simulink model "Key_signal_process"  (R2021a)
settings: configuration reference "AION_IDS_Speedgoat" (kept outside this file)
undefined symbols (not defined in the file): original_value_current, original_value_previous, original_value_queue, processed_value_current, processed_value_previous, processed_value_queue, refitted_value_current, refitted_value_previous, refitted_value_queue, Validation
libraries: simulink x5
settings Model: DataDictionary=Key_Signal_Process.sldd  Creator=xinrui  LastModifiedBy=Administrator
settings ConfigSetRef: SourceName=AION_IDS_Speedgoat

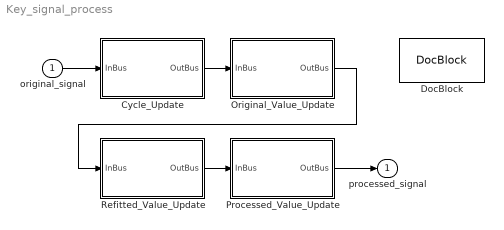
== system Key_signal_process ==
  original_signal : Inport  OutDataTypeStr=Bus: Key_Signal_Info  PortDimensions=1
  Cycle_Update : Subsystem
  DocBlock : simulink/Model-Wide Utilities/DocBlock  DocumentType=HTML  mask(DocBlock){}
      mask Display:
      | plot([.8 0 0 1 1 .8 .8 1],[1 1 0 0 .8 1 .8 .8]);
      | text(.5,.6,'CHANGELOG','horizontalalignment','center');
      | text(.95,.05,get_param(gcb,'DocumentType'),'verticalalignment','bottom','horizontalalignment','right');
  Original_Value_Update : Subsystem
  Processed_Value_Update : Subsystem
  Refitted_Value_Update : Subsystem
  processed_signal : Outport  OutDataTypeStr=Bus: Key_Signal_Info  PortDimensions=1
  wires:
  Refitted_Value_Update/1(OutBus) -> Processed_Value_Update/1(InBus)
  Original_Value_Update/1(OutBus) -> Refitted_Value_Update/1(InBus)
  original_signal/1 -> Cycle_Update/1(InBus)
  Processed_Value_Update/1(OutBus) -> processed_signal/1
  Cycle_Update/1(OutBus) -> Original_Value_Update/1(InBus)

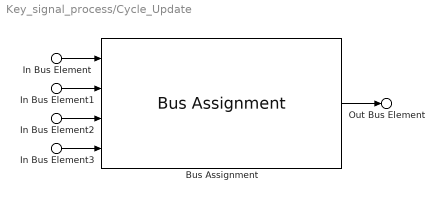
== system Key_signal_process/Cycle_Update ==
  In Bus Element : Inport  PortName=InBus
  In Bus Element1 : Inport  PortName=InBus  Element=original_value_current
  In Bus Element2 : Inport  PortName=InBus  Element=refitted_value_current
  In Bus Element3 : Inport  PortName=InBus  Element=processed_value_current
  Bus Assignment : BusAssignment  AssignedSignals=original_value_previous,refitted_value_previous,processed_value_previous
  Out Bus Element : Outport  PortName=OutBus
  wires:
  Bus Assignment/1 -> Out Bus Element/1
  In Bus Element1/1 -> Bus Assignment/2
  In Bus Element2/1 -> Bus Assignment/3
  In Bus Element3/1 -> Bus Assignment/4
  In Bus Element/1 -> Bus Assignment/1

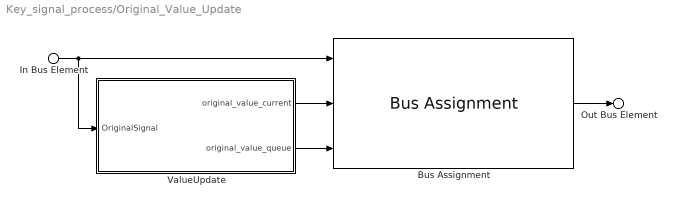
== system Key_signal_process/Original_Value_Update ==
  In Bus Element : Inport  PortName=InBus
  Bus Assignment : BusAssignment  AssignedSignals=original_value_current,original_value_queue
  ValueUpdate : Subsystem
  Out Bus Element : Outport  PortName=OutBus
  wires:
  In Bus Element/1 -> ValueUpdate/1(OriginalSignal), Bus Assignment/1
  ValueUpdate/2(original_value_queue) -> Bus Assignment/3
  ValueUpdate/1(original_value_current) -> Bus Assignment/2
  Bus Assignment/1 -> Out Bus Element/1

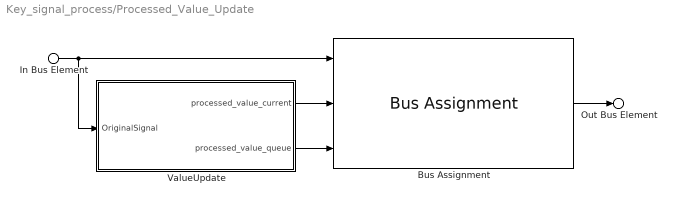
== system Key_signal_process/Processed_Value_Update ==
  In Bus Element : Inport  PortName=InBus
  Bus Assignment : BusAssignment  AssignedSignals=processed_value_current,processed_value_queue
  ValueUpdate : Subsystem
  Out Bus Element : Outport  PortName=OutBus
  wires:
  In Bus Element/1 -> Bus Assignment/1, ValueUpdate/1(OriginalSignal)
  ValueUpdate/2(processed_value_queue) -> Bus Assignment/3
  ValueUpdate/1(processed_value_current) -> Bus Assignment/2
  Bus Assignment/1 -> Out Bus Element/1

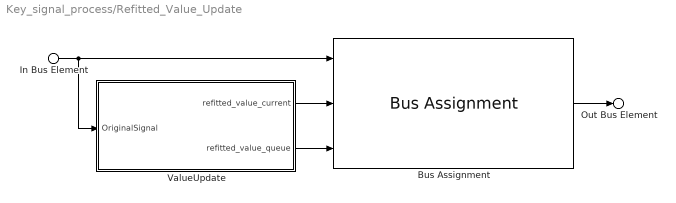
== system Key_signal_process/Refitted_Value_Update ==
  In Bus Element : Inport  PortName=InBus
  Bus Assignment : BusAssignment  AssignedSignals=refitted_value_current,refitted_value_queue
  ValueUpdate : Subsystem
  Out Bus Element : Outport  PortName=OutBus
  wires:
  Bus Assignment/1 -> Out Bus Element/1
  ValueUpdate/1(refitted_value_current) -> Bus Assignment/2
  ValueUpdate/2(refitted_value_queue) -> Bus Assignment/3
  In Bus Element/1 -> Bus Assignment/1, ValueUpdate/1(OriginalSignal)

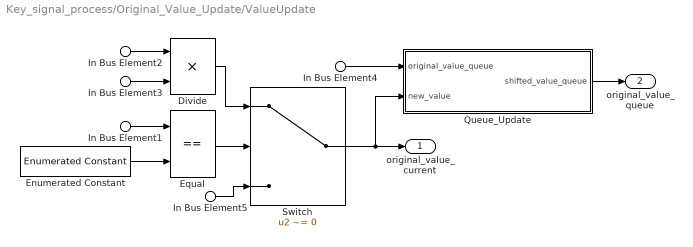
== system Key_signal_process/Original_Value_Update/ValueUpdate ==
  In Bus Element2 : Inport  PortName=OriginalSignal  Element=input_value
  In Bus Element1 : Inport  PortName=OriginalSignal  Element=input_value_lock
  In Bus Element5 : Inport  PortName=OriginalSignal  Element=original_value_previous
  In Bus Element4 : Inport  PortName=OriginalSignal  Element=original_value_queue
  In Bus Element3 : Inport  PortName=OriginalSignal  Element=unit_converter_factor
  Divide : Product  Inputs=**  OutDataTypeStr=double
  Enumerated Constant : simulink/Sources/Enumerated Constant  OutDataTypeStr=Enum: Validation  Value=Validation.Invalid  SampleTime=-1
  Equal : RelationalOperator  Operator===  OutDataTypeStr=boolean  RndMeth=Simplest
  Queue_Update : Subsystem
  Switch : Switch  Criteria=u2 ~= 0  OutDataTypeStr=double
  original_value_current : Outport  OutDataTypeStr=double  PortDimensions=1
  original_value_queue : Outport  Port=2  OutDataTypeStr=double
  wires:
  Switch/1 -> Queue_Update/2(new_value), original_value_current/1
  In Bus Element1/1 -> Equal/1
  Equal/1 -> Switch/2
  In Bus Element3/1 -> Divide/2
  In Bus Element2/1 -> Divide/1
  In Bus Element4/1 -> Queue_Update/1(original_value_queue)
  Divide/1 -> Switch/1
  Enumerated Constant/1 -> Equal/2
  Queue_Update/1(shifted_value_queue) -> original_value_queue/1
  In Bus Element5/1 -> Switch/3

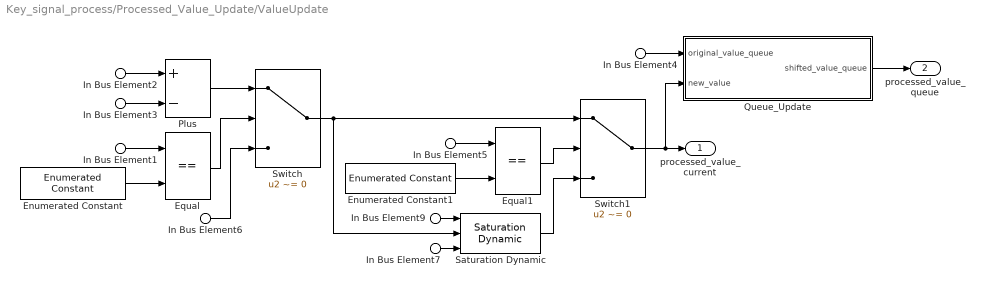
== system Key_signal_process/Processed_Value_Update/ValueUpdate ==
  In Bus Element4 : Inport  PortName=OriginalSignal  Element=original_value_queue
  In Bus Element2 : Inport  PortName=OriginalSignal  Element=refitted_value_current
  In Bus Element1 : Inport  PortName=OriginalSignal  Element=processed_value_lock
  In Bus Element6 : Inport  PortName=OriginalSignal  Element=processed_value_previous
  In Bus Element3 : Inport  PortName=OriginalSignal  Element=value_offset
  In Bus Element5 : Inport  PortName=OriginalSignal  Element=absolute_amplitude_limit_mode
  In Bus Element9 : Inport  PortName=OriginalSignal  Element=max_value
  In Bus Element7 : Inport  PortName=OriginalSignal  Element=min_value
  Enumerated Constant : simulink/Sources/Enumerated Constant  OutDataTypeStr=Enum: Validation  Value=Validation.Invalid  SampleTime=-1
  Enumerated Constant1 : simulink/Sources/Enumerated Constant  OutDataTypeStr=Enum: Validation  Value=Validation.Invalid  SampleTime=-1
  Equal : RelationalOperator  Operator===  OutDataTypeStr=boolean  RndMeth=Simplest
  Equal1 : RelationalOperator  Operator===  OutDataTypeStr=boolean  RndMeth=Simplest
  Plus : Sum  Inputs=+-  OutDataTypeStr=double
  Queue_Update : Subsystem
  Saturation Dynamic : simulink/Discontinuities/Saturation Dynamic  OutMin=[]  OutMax=[]  OutDataTypeStr=double  OutputDataTypeScalingMode=double  OutDataType=fixdt(1, 16)  OutScaling=2^-10  DoSatur=off
  Switch : Switch  Criteria=u2 ~= 0  OutDataTypeStr=double
  Switch1 : Switch  Criteria=u2 ~= 0  OutDataTypeStr=double
  processed_value_current : Outport  OutDataTypeStr=double  PortDimensions=1
  processed_value_queue : Outport  Port=2  OutDataTypeStr=double
  wires:
  Switch/1 -> Saturation Dynamic/2, Switch1/1
  Plus/1 -> Switch/1
  In Bus Element2/1 -> Plus/1
  Equal/1 -> Switch/2
  Saturation Dynamic/1 -> Switch1/3
  In Bus Element3/1 -> Plus/2
  In Bus Element5/1 -> Equal1/1
  Enumerated Constant1/1 -> Equal1/2
  Switch1/1 -> Queue_Update/2(new_value), processed_value_current/1
  Enumerated Constant/1 -> Equal/2
  Equal1/1 -> Switch1/2
  In Bus Element6/1 -> Switch/3
  In Bus Element1/1 -> Equal/1
  Queue_Update/1(shifted_value_queue) -> processed_value_queue/1
  In Bus Element4/1 -> Queue_Update/1(original_value_queue)
  In Bus Element7/1 -> Saturation Dynamic/3
  In Bus Element9/1 -> Saturation Dynamic/1

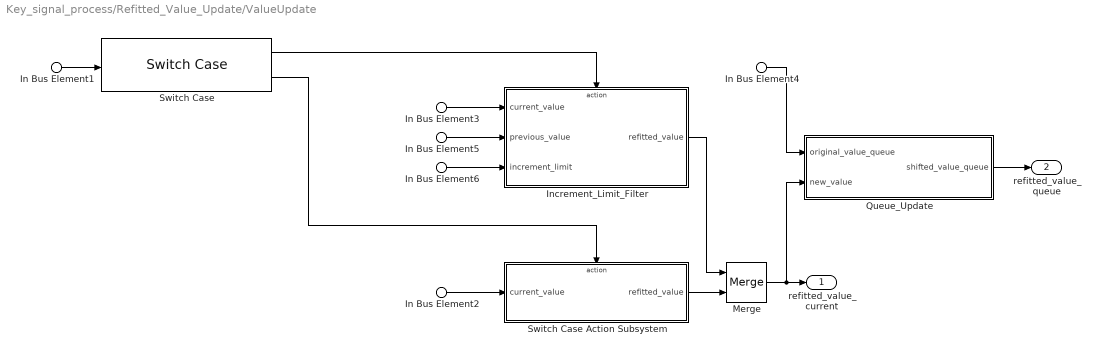
== system Key_signal_process/Refitted_Value_Update/ValueUpdate ==
  In Bus Element2 : Inport  PortName=OriginalSignal  Element=original_value_current
  In Bus Element3 : Inport  PortName=OriginalSignal  Element=original_value_current
  In Bus Element5 : Inport  PortName=OriginalSignal  Element=refitted_value_previous
  In Bus Element4 : Inport  PortName=OriginalSignal  Element=refitted_value_queue
  In Bus Element1 : Inport  PortName=OriginalSignal  Element=processing_mode
  In Bus Element6 : Inport  PortName=OriginalSignal  Element=increment_limit
  Increment_Limit_Filter : Subsystem  TreatAsAtomicUnit=on
  Merge : Merge
  Queue_Update : Subsystem
  Switch Case : SwitchCase  CaseConditions={SignalProcessingMode.IncrementLimitFilter}
  Switch Case Action Subsystem : Subsystem  TreatAsAtomicUnit=on
  refitted_value_current : Outport  OutDataTypeStr=double  PortDimensions=1
  refitted_value_queue : Outport  Port=2  OutDataTypeStr=double
  wires:
  In Bus Element6/1 -> Increment_Limit_Filter/3(increment_limit)
  In Bus Element2/1 -> Switch Case Action Subsystem/1(current_value)
  Switch Case Action Subsystem/1(refitted_value) -> Merge/2
  Increment_Limit_Filter/1(refitted_value) -> Merge/1
  Switch Case/1 -> Increment_Limit_Filter/Action
  Merge/1 -> refitted_value_current/1, Queue_Update/2(new_value)
  In Bus Element1/1 -> Switch Case/1
  In Bus Element3/1 -> Increment_Limit_Filter/1(current_value)
  Queue_Update/1(shifted_value_queue) -> refitted_value_queue/1
  In Bus Element4/1 -> Queue_Update/1(original_value_queue)
  Switch Case/2 -> Switch Case Action Subsystem/Action
  In Bus Element5/1 -> Increment_Limit_Filter/2(previous_value)

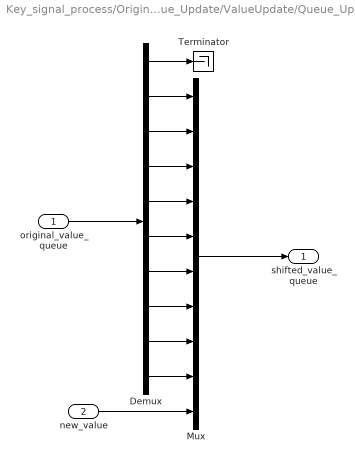
== system Key_signal_process/Original_Value_Update/ValueUpdate/Queue_Update ==
  original_value_queue : Inport  OutDataTypeStr=double
  new_value : Inport  Port=2  OutDataTypeStr=double  PortDimensions=1
  Demux : Demux  Outputs=10
  Mux : Mux  Inputs=10
  Terminator : Terminator
  shifted_value_queue : Outport  OutDataTypeStr=double
  wires:
  original_value_queue/1 -> Demux/1
  Demux/8 -> Mux/7
  Demux/10 -> Mux/9
  Demux/5 -> Mux/4
  Demux/2 -> Mux/1
  Mux/1 -> shifted_value_queue/1
  Demux/1 -> Terminator/1
  Demux/7 -> Mux/6
  Demux/3 -> Mux/2
  Demux/6 -> Mux/5
  new_value/1 -> Mux/10
  Demux/4 -> Mux/3
  Demux/9 -> Mux/8

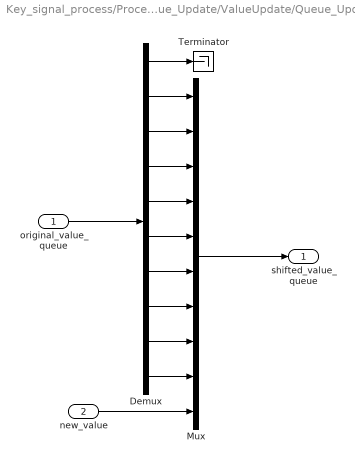
== system Key_signal_process/Processed_Value_Update/ValueUpdate/Queue_Update ==
  original_value_queue : Inport  OutDataTypeStr=double
  new_value : Inport  Port=2  OutDataTypeStr=double  PortDimensions=1
  Demux : Demux  Outputs=10
  Mux : Mux  Inputs=10
  Terminator : Terminator
  shifted_value_queue : Outport  OutDataTypeStr=double
  wires:
  original_value_queue/1 -> Demux/1
  Demux/8 -> Mux/7
  Demux/10 -> Mux/9
  Demux/5 -> Mux/4
  Demux/2 -> Mux/1
  Mux/1 -> shifted_value_queue/1
  Demux/1 -> Terminator/1
  Demux/7 -> Mux/6
  Demux/3 -> Mux/2
  Demux/6 -> Mux/5
  new_value/1 -> Mux/10
  Demux/4 -> Mux/3
  Demux/9 -> Mux/8

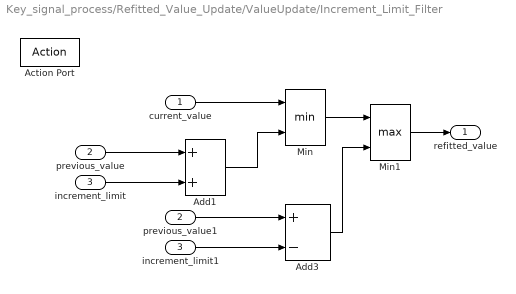
== system Key_signal_process/Refitted_Value_Update/ValueUpdate/Increment_Limit_Filter ==
  current_value : Inport  OutDataTypeStr=double  PortDimensions=1
  previous_value : Inport  Port=2  OutDataTypeStr=double  PortDimensions=1
  increment_limit : Inport  Port=3  OutDataTypeStr=double  PortDimensions=1
  Action Port : ActionPort  ActionPortLabel=case [ IncrementLimitFilter ]:
  Add1 : Sum  OutDataTypeStr=double
  Add3 : Sum  Inputs=+-  OutDataTypeStr=double
  Min : MinMax  Inputs=2  OutDataTypeStr=double
  Min1 : MinMax  Function=max  Inputs=2  OutDataTypeStr=double
  increment_limit1 : InportShadow  Port=3  OutDataTypeStr=double  PortDimensions=1
  previous_value1 : InportShadow  Port=2  OutDataTypeStr=double  PortDimensions=1
  refitted_value : Outport  OutDataTypeStr=double  PortDimensions=1
  wires:
  previous_value1/1 -> Add3/1
  increment_limit/1 -> Add1/2
  Min/1 -> Min1/1
  increment_limit1/1 -> Add3/2
  current_value/1 -> Min/1
  Add1/1 -> Min/2
  Min1/1 -> refitted_value/1
  Add3/1 -> Min1/2
  previous_value/1 -> Add1/1

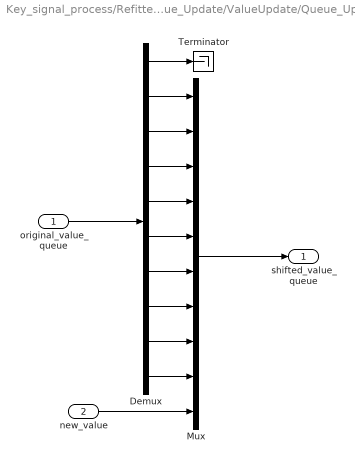
== system Key_signal_process/Refitted_Value_Update/ValueUpdate/Queue_Update ==
  original_value_queue : Inport  OutDataTypeStr=double
  new_value : Inport  Port=2  OutDataTypeStr=double  PortDimensions=1
  Demux : Demux  Outputs=10
  Mux : Mux  Inputs=10
  Terminator : Terminator
  shifted_value_queue : Outport  OutDataTypeStr=double
  wires:
  original_value_queue/1 -> Demux/1
  Demux/8 -> Mux/7
  Demux/10 -> Mux/9
  Demux/5 -> Mux/4
  Demux/2 -> Mux/1
  Mux/1 -> shifted_value_queue/1
  Demux/1 -> Terminator/1
  Demux/7 -> Mux/6
  Demux/3 -> Mux/2
  Demux/6 -> Mux/5
  new_value/1 -> Mux/10
  Demux/4 -> Mux/3
  Demux/9 -> Mux/8

== system Key_signal_process/Refitted_Value_Update/ValueUpdate/Switch Case Action Subsystem ==
  current_value : Inport  OutDataTypeStr=double  PortDimensions=1
  Action Port : ActionPort  ActionPortLabel=default:
  Signal Copy : SignalConversion  OverrideOpt=off
  refitted_value : Outport  OutDataTypeStr=double  PortDimensions=1
  wires:
  current_value/1 -> Signal Copy/1
  Signal Copy/1 -> refitted_value/1
